simulink model "course_hold_AP_2e"  (R2015a)
settings: Solver=ode45  SolverMode=SingleTasking  StartTime=0.0  StopTime=600  RelTol=1e-3
values from neighbouring files (symbols this model uses):
  g = 9.81    [Problem3.m]
  kd_fi = (2*zeta_fi*omega_fi-alpha_fi1)/alpha_fi2    [Problem3.m]
  ki_chi = omega_chi^2*V_g/g    [Problem3.m]
  ki_fi = -0    (= 0)    [Problem3.m]
  kp_chi = 2*zeta_chi*omega_chi*V_g/g    [Problem3.m]
  kp_fi = -2    [Problem3.m]
  V_g = 580/3.6    (= 161.111111111)    [Problem3.m]
libraries: simulink_extras x2
settings Model: CovMetricSettings=dwe  CovHtmlReporting=off  covSaveCumulativeToWorkspaceVar=off  CovSaveSingleToWorkspaceVar=off  CovExternalEMLEnable=on  Creator=marti  LastModifiedBy=Anders Vagle
settings DataIOCC: LimitDataPoints=off  SaveFormat=Dataset
settings DebuggingCC: SFUnexpectedBacktrackingDiag=error  SFNoUnconditionalDefaultTransitionDiag=error
settings HardwareCC: ProdBitPerPointer=64  ProdLargestAtomicFloat=Float  ProdIntDivRoundTo=Zero  ProdEndianess=LittleEndian  ProdHWDeviceType=Specified
settings ModelReferenceCC: PropagateSignalLabelsOutOfModel=on
settings GRTTargetCC: TargetLangStandard=C99 (ISO)  GeneratePreprocessorConditionals=Use local settings

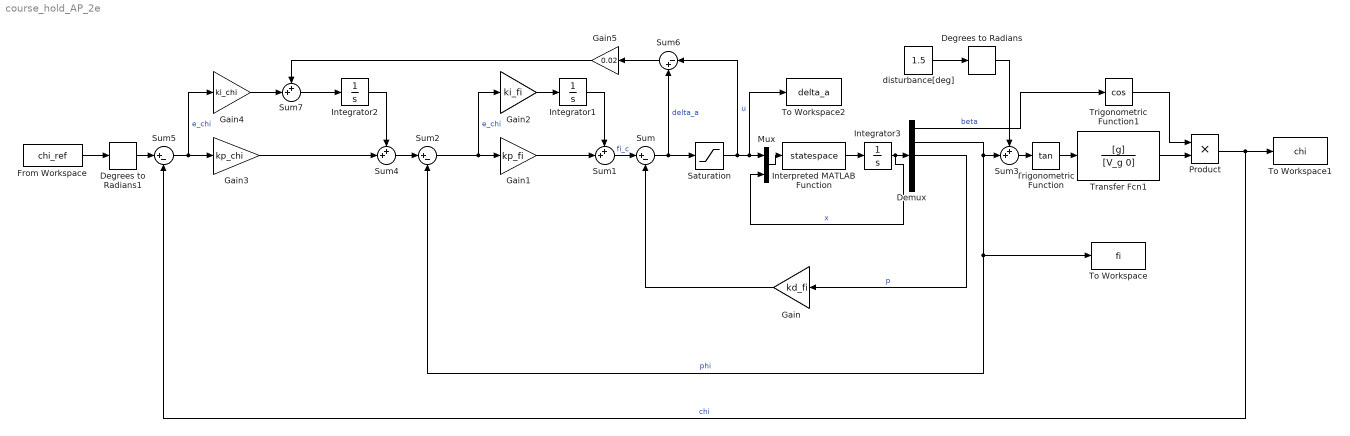
== system course_hold_AP_2e ==
  Degrees to Radians : simulink_extras/Transformations/Degrees to Radians
  Degrees to Radians1 : simulink_extras/Transformations/Degrees to Radians
  Demux : Demux  Outputs=5
  From Workspace : FromWorkspace  VariableName=chi_ref  SampleTime=0  Interpolate=off  OutputAfterFinalValue=Holding final value
  Gain : Gain  Gain=kd_fi
  Gain1 : Gain  Gain=kp_fi
  Gain2 : Gain  Gain=ki_fi
  Gain3 : Gain  Gain=kp_chi
  Gain4 : Gain  Gain=ki_chi
  Gain5 : Gain  Gain=0.02
  Integrator1 : Integrator
  Integrator2 : Integrator
  Integrator3 : Integrator
  Interpreted MATLAB Function : MATLABFcn  MATLABFcn=statespace  OutputDimensions=5  OutputSignalType=real
  Mux : Mux  Inputs=2
  Product : Product
  Saturation : Saturate  UpperLimit=30/180*pi  LowerLimit=-30/180*pi
  Sum : Sum  Inputs=|+-
  Sum{1,3..4,7} (4 alike) : Sum  Inputs=++|
  Sum2 : Sum  Inputs=|+-
  Sum5 : Sum  Inputs=|+-
  Sum6 : Sum  Inputs=|-+
  To Workspace : ToWorkspace  VariableName=fi  SaveFormat=Timeseries  SampleTime=-1
  To Workspace1 : ToWorkspace  VariableName=chi  SaveFormat=Timeseries  SampleTime=-1
  To Workspace2 : ToWorkspace  VariableName=delta_a  SaveFormat=Timeseries  SampleTime=-1
  Transfer Fcn1 : TransferFcn  Numerator=[g]  Denominator=[V_g 0]
  Trigonometric Function : Trigonometry  Operator=tan
  Trigonometric Function1 : Trigonometry  Operator=cos
  disturbance[deg] : Constant  Value=1.5
  wires:
  Gain/1 -> Sum/2
  Sum1/1 -> Sum/1  "fi_c"
  Integrator1/1 -> Sum1/1
  Gain1/1 -> Sum1/2
  Sum2/1 -> Gain2/1, Gain1/1  "e_chi"
  Demux/2 -> Sum2/2, To Workspace/1, Sum3/2  "phi"
  Integrator2/1 -> Sum4/1
  Gain3/1 -> Sum4/2
  Sum5/1 -> Gain4/1, Gain3/1  "e_chi"
  Sum/1 -> Saturation/1, Sum6/2  "delta_a"
  Sum4/1 -> Sum2/1
  Degrees to Radians1/1 -> Sum5/1
  disturbance[deg]/1 -> Degrees to Radians/1
  Degrees to Radians/1 -> Sum3/1
  From Workspace/1 -> Degrees to Radians1/1
  Sum3/1 -> Trigonometric Function/1
  Trigonometric Function/1 -> Transfer Fcn1/1
  Demux/1 -> Trigonometric Function1/1  "beta"
  Transfer Fcn1/1 -> Product/2
  Trigonometric Function1/1 -> Product/1
  Product/1 -> To Workspace1/1, Sum5/2  "chi"
  Saturation/1 -> Sum6/1, Mux/1, To Workspace2/1  "u"
  Interpreted MATLAB Function/1 -> Integrator3/1
  Integrator3/1 -> Mux/2, Demux/1  "x"
  Demux/3 -> Gain/1  "p"
  Mux/1 -> Interpreted MATLAB Function/1
  Sum6/1 -> Gain5/1
  Gain2/1 -> Integrator1/1
  Gain4/1 -> Sum7/2
  Sum7/1 -> Integrator2/1
  Gain5/1 -> Sum7/1
